simulink model "Regen"  (R2016b)
settings: Solver=VariableStepAuto  StartTime=0.0  StopTime=100  RelTol=1e-3
values from neighbouring files (symbols this model uses):
  alpha = mean(alpha)    [systemident.m]
  C = 10    [RUN.m]
  N =     [Gear Ratios.mat]
  R = mean(R)    [systemident.m]
settings Model: Creator=R4hul  LastModifiedBy=R4hul

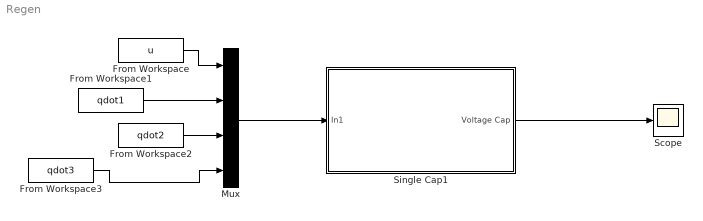
== system Regen ==
  From Workspace : FromWorkspace  VariableName=u  SampleTime=0
  From Workspace1 : FromWorkspace  VariableName=qdot1  SampleTime=0
  From Workspace2 : FromWorkspace  VariableName=qdot2  SampleTime=0
  From Workspace3 : FromWorkspace  VariableName=qdot3  SampleTime=0
  Mux : Mux
  Scope : Scope
  Single Cap1 : Subsystem
  wires:
  From Workspace/1 -> Mux/1
  From Workspace1/1 -> Mux/2
  From Workspace2/1 -> Mux/3
  From Workspace3/1 -> Mux/4
  Mux/1 -> Single Cap1/1(In1)
  Single Cap1/1(Voltage Cap) -> Scope/1

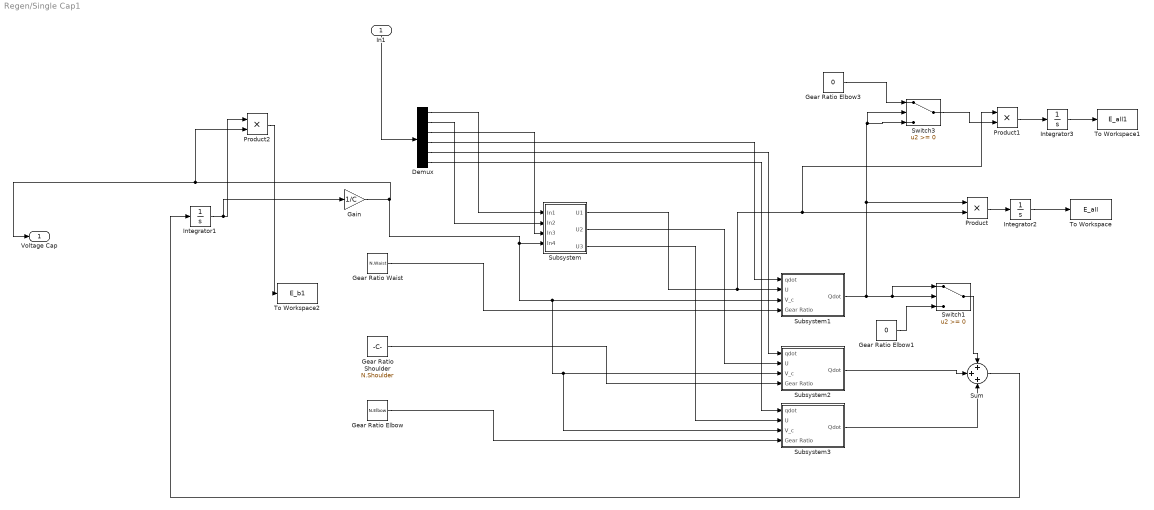
== system Regen/Single Cap1 ==
  In1 : Inport
  Demux : Demux  Outputs=6
  Gain : Gain  Gain=1/C
  Gear Ratio Elbow : Constant  Value=N.Elbow
  Gear Ratio Elbow1 : Constant  Value=0
  Gear Ratio Elbow3 : Constant  Value=0
  "Gear Ratio Shoulder " : Constant  Value=N.Shoulder
  Gear Ratio Waist : Constant  Value=N.Waist
  Integrator1 : Integrator  InitialCondition=C*30
  Integrator2 : Integrator
  Integrator3 : Integrator
  Product : Product
  Product1 : Product
  Product2 : Product
  Subsystem : Subsystem
  Subsystem1 : Subsystem
  Subsystem2 : Subsystem
  Subsystem3 : Subsystem
  Sum : Sum  Inputs=3
  Switch1 : Switch
  Switch3 : Switch
  To Workspace : ToWorkspace  VariableName=E_all  SampleTime=-1
  To Workspace1 : ToWorkspace  VariableName=E_all1  SampleTime=-1
  To Workspace2 : ToWorkspace  VariableName=E_b1  SampleTime=-1
  Voltage Cap : Outport
  wires:
  Demux/6 -> Subsystem3/1(qdot)
  Demux/5 -> Subsystem2/1(qdot)
  Demux/4 -> Subsystem1/1(qdot)
  Demux/3 -> Subsystem/3(In3)
  Demux/2 -> Subsystem/2(In2)
  Demux/1 -> Subsystem/1(In1)
  In1/1 -> Demux/1
  Gain/1 -> Product2/2, Voltage Cap/1, Subsystem1/3(V_c), Subsystem2/3(V_c), Subsystem3/3(V_c), Subsystem/4(In4)
  "Gear Ratio Shoulder "/1 -> Subsystem2/4(Gear Ratio)
  Gear Ratio Elbow/1 -> Subsystem3/4(Gear Ratio)
  Subsystem2/1(Qdot) -> Sum/2
  Subsystem/3(U3) -> Subsystem3/2(U)
  Subsystem/1(U1) -> Subsystem1/2(U), Product1/1, Product/2
  Gear Ratio Waist/1 -> Subsystem1/4(Gear Ratio)
  Subsystem/2(U2) -> Subsystem2/2(U)
  Subsystem3/1(Qdot) -> Sum/3
  Sum/1 -> Integrator1/1
  Subsystem1/1(Qdot) -> Product/1, Switch3/3, Switch3/2, Switch1/1, Switch1/2
  Switch1/1 -> Sum/1
  Gear Ratio Elbow1/1 -> Switch1/3
  Product/1 -> Integrator2/1
  Integrator2/1 -> To Workspace/1
  Gear Ratio Elbow3/1 -> Switch3/1
  Product1/1 -> Integrator3/1
  Integrator3/1 -> To Workspace1/1
  Switch3/1 -> Product1/2
  Product2/1 -> To Workspace2/1
  Integrator1/1 -> Gain/1, Product2/1

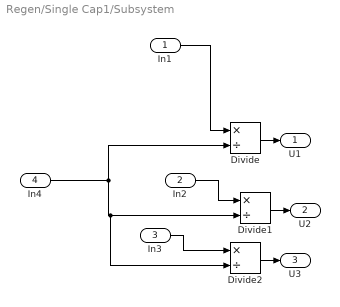
== system Regen/Single Cap1/Subsystem ==
  In1 : Inport
  In2 : Inport  Port=2
  In3 : Inport  Port=3
  In4 : Inport  Port=4
  Divide : Product  Inputs=*/
  Divide1 : Product  Inputs=*/
  Divide2 : Product  Inputs=*/
  U1 : Outport
  U2 : Outport  Port=2
  U3 : Outport  Port=3
  wires:
  In4/1 -> Divide/2, Divide1/2, Divide2/2
  In3/1 -> Divide2/1
  In2/1 -> Divide1/1
  In1/1 -> Divide/1
  Divide/1 -> U1/1
  Divide1/1 -> U2/1
  Divide2/1 -> U3/1

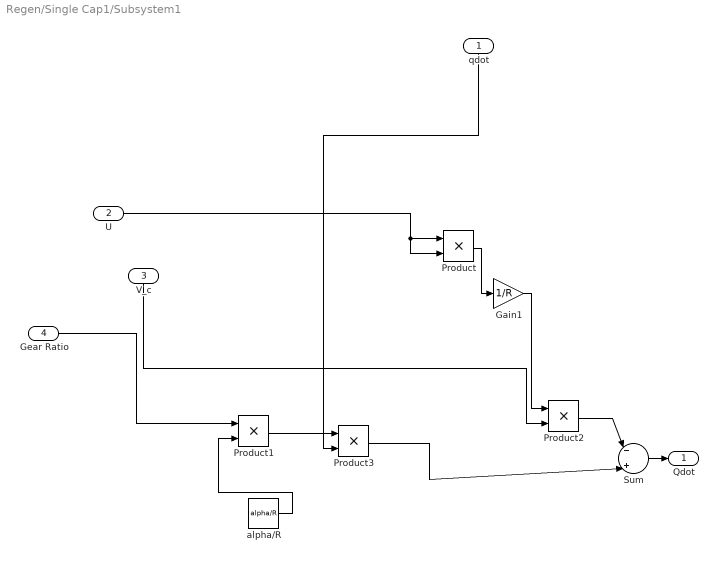
== system Regen/Single Cap1/Subsystem1 ==
  qdot : Inport
  U : Inport  Port=2
  V_c : Inport  Port=3
  Gear Ratio : Inport  Port=4
  Gain1 : Gain  Gain=1/R
  Product{,1..3} (4 alike) : Product
  Sum : Sum  Inputs=|-|+|
  alpha/R : Constant  Value=alpha/R
  Qdot : Outport
  wires:
  Gear Ratio/1 -> Product1/1
  Gain1/1 -> Product2/1
  Product1/1 -> Product3/1
  Product3/1 -> Sum/2
  U/1 -> Product/1, Product/2
  Product/1 -> Gain1/1
  alpha/R/1 -> Product1/2
  Sum/1 -> Qdot/1
  V_c/1 -> Product2/2
  qdot/1 -> Product3/2
  Product2/1 -> Sum/1

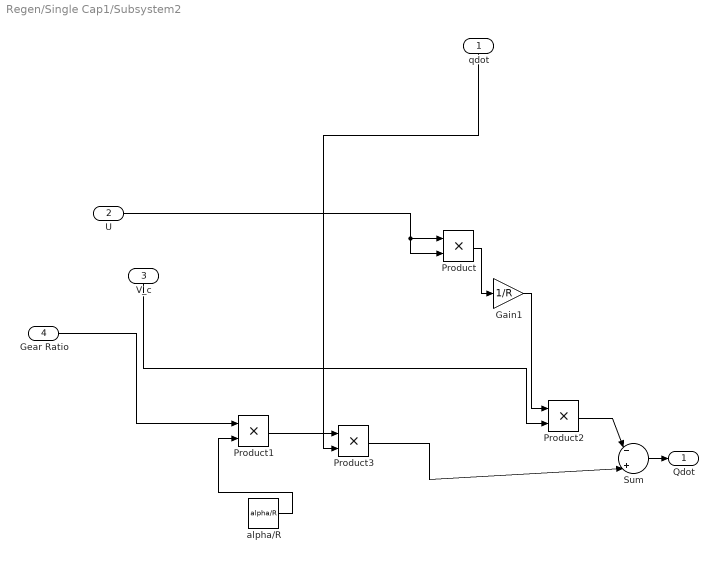
== system Regen/Single Cap1/Subsystem2 ==
  qdot : Inport
  U : Inport  Port=2
  V_c : Inport  Port=3
  Gear Ratio : Inport  Port=4
  Gain1 : Gain  Gain=1/R
  Product{,1..3} (4 alike) : Product
  Sum : Sum  Inputs=|-|+|
  alpha/R : Constant  Value=alpha/R
  Qdot : Outport
  wires:
  Product2/1 -> Sum/1
  qdot/1 -> Product3/2
  V_c/1 -> Product2/2
  Sum/1 -> Qdot/1
  alpha/R/1 -> Product1/2
  Product/1 -> Gain1/1
  U/1 -> Product/2, Product/1
  Product3/1 -> Sum/2
  Product1/1 -> Product3/1
  Gain1/1 -> Product2/1
  Gear Ratio/1 -> Product1/1

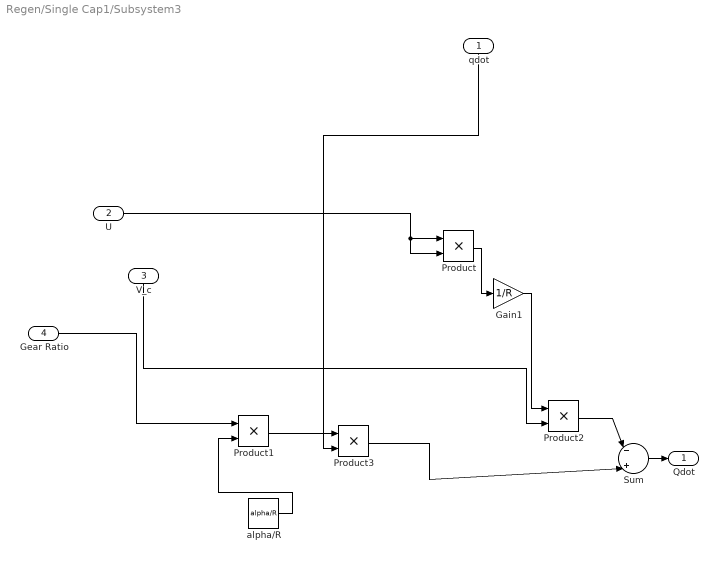
== system Regen/Single Cap1/Subsystem3 ==
  qdot : Inport
  U : Inport  Port=2
  V_c : Inport  Port=3
  Gear Ratio : Inport  Port=4
  Gain1 : Gain  Gain=1/R
  Product{,1..3} (4 alike) : Product
  Sum : Sum  Inputs=|-|+|
  alpha/R : Constant  Value=alpha/R
  Qdot : Outport
  wires:
  Gear Ratio/1 -> Product1/1
  Gain1/1 -> Product2/1
  Product1/1 -> Product3/1
  Product3/1 -> Sum/2
  U/1 -> Product/1, Product/2
  Product/1 -> Gain1/1
  alpha/R/1 -> Product1/2
  Sum/1 -> Qdot/1
  V_c/1 -> Product2/2
  qdot/1 -> Product3/2
  Product2/1 -> Sum/1
